simulink model "TV"  (R2025b)
settings: Solver=VariableStepAuto  StartTime=0.0  StopTime=10.0  RelTol=1e-3
undefined symbols (not defined in the file): tv
Description:
  | Adapted De Novellis et al. (IEEE TVT 2014) feedforward + PID TV controller.
settings Model: Creator=jaiden  LastModifiedBy=jaiden

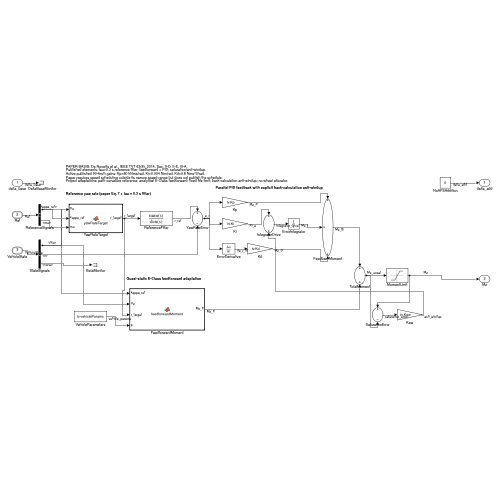
[thumbnail: Simulink's stored preview of the top-level diagram]
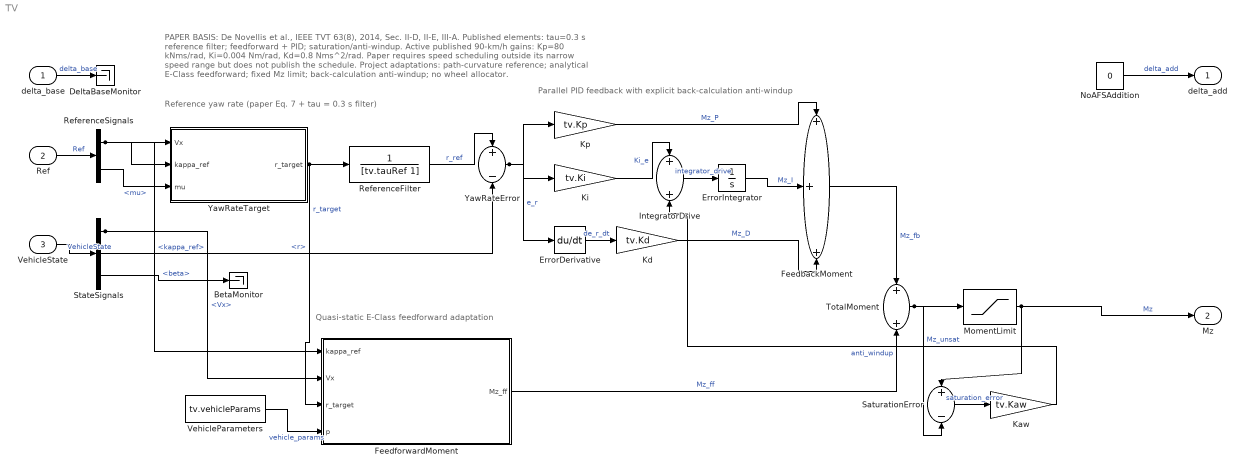
== system TV ==
  note: PAPER BASIS: De Novellis et al., IEEE TVT 63(8), 2014, Sec. II-D, II-E, III-A.
      | Published elements: tau=0.3 s reference filter; feedforward + PID; saturation/anti-windup.
      | Active published 90-km/h gains: Kp=80 kNms/rad, Ki=0.004 Nm/rad, Kd=0.8 Nms^2/rad.
      | Paper requires speed scheduling outside its narrow speed range but does not publish the schedule.
      | Project adaptations: path-curvature reference; analytical E-Class feedforward; fixed Mz limit; back-calculation anti-windup; no wheel allocator.
  note: Reference yaw rate (paper Eq. 7 + tau = 0.3 s filter)
  note: Parallel PID feedback with explicit back-calculation anti-windup
  note: Quasi-static E-Class feedforward adaptation
  delta_base : Inport
  Ref : Inport  Port=2  OutDataTypeStr=Bus: ReferenceBus
  VehicleState : Inport  Port=3  OutDataTypeStr=Bus: VehicleStateBus
  BetaMonitor : Terminator
  DeltaBaseMonitor : Terminator
  ErrorDerivative : Derivative
  ErrorIntegrator : Integrator
  FeedbackMoment : Sum  Inputs=+++
  FeedforwardMoment : MATLAB Function  TreatAsAtomicUnit=on
  IntegratorDrive : Sum  Description=Integral drive = Ki*e_r + Kaw*(Mz-Mz_unsat). The paper states
  Kaw : Gain  Description=Project-specific back-calculation gain. The paper confirms  Gain=tv.Kaw
  Kd : Gain  Gain=tv.Kd
  Ki : Gain  Gain=tv.Ki
  Kp : Gain  Gain=tv.Kp
  MomentLimit : Saturate  Description=Fixed bicycle-model yaw-moment authority; replace with plant-specific  UpperLimit=tv.MzMax  LowerLimit=-tv.MzMax  ZeroCross=off
  NoAFSAddition : Constant  Value=0
  ReferenceFilter : TransferFcn  Description=Paper Sec. II-D: first-order reference-yaw-rate factor, tau = 0.3 s.  Numerator=1  Denominator=[tv.tauRef 1]
  ReferenceSignals : BusSelector  OutputSignals=kappa_ref,mu
  SaturationError : Sum  Inputs=+-
  StateSignals : BusSelector  OutputSignals=Vx,r,beta
  TotalMoment : Sum
  VehicleParameters : Constant  Description=[m, a, b, Caf, Car] for analytical E-Class feedforward.  Value=tv.vehicleParams
  YawRateError : Sum  Description=e_r = r_ref - r matches negative feedback in paper Eq. (5) and  Inputs=+-
  YawRateTarget : MATLAB Function  TreatAsAtomicUnit=on
  delta_add : Outport
  Mz : Outport  Port=2
  wires:
  NoAFSAddition/1 -> delta_add/1  "delta_add"
  delta_base/1 -> DeltaBaseMonitor/1  "delta_base"
  Ref/1 -> ReferenceSignals/1  "Ref"
  VehicleState/1 -> StateSignals/1  "VehicleState"
  StateSignals/3 -> BetaMonitor/1  "<beta>"
  ReferenceSignals/1 -> YawRateTarget/2(kappa_ref), FeedforwardMoment/1(kappa_ref)  "<kappa_ref>"
  ReferenceSignals/2 -> YawRateTarget/3(mu)  "<mu>"
  StateSignals/1 -> YawRateTarget/1(Vx), FeedforwardMoment/2(Vx)  "<Vx>"
  YawRateTarget/1(r_target) -> ReferenceFilter/1, FeedforwardMoment/3(r_target)  "r_target"
  ReferenceFilter/1 -> YawRateError/1  "r_ref"
  StateSignals/2 -> YawRateError/2  "<r>"
  YawRateError/1 -> Kp/1, Ki/1, ErrorDerivative/1  "e_r"
  Ki/1 -> IntegratorDrive/1  "Ki_e"
  IntegratorDrive/1 -> ErrorIntegrator/1  "integrator_drive"
  ErrorDerivative/1 -> Kd/1  "de_r_dt"
  Kp/1 -> FeedbackMoment/1  "Mz_P"
  ErrorIntegrator/1 -> FeedbackMoment/2  "Mz_I"
  Kd/1 -> FeedbackMoment/3  "Mz_D"
  VehicleParameters/1 -> FeedforwardMoment/4(p)  "vehicle_params"
  FeedbackMoment/1 -> TotalMoment/1  "Mz_fb"
  FeedforwardMoment/1(Mz_ff) -> TotalMoment/2  "Mz_ff"
  TotalMoment/1 -> MomentLimit/1, SaturationError/2  "Mz_unsat"
  MomentLimit/1 -> Mz/1, SaturationError/1  "Mz"
  SaturationError/1 -> Kaw/1  "saturation_error"
  Kaw/1 -> IntegratorDrive/2  "anti_windup"

== matlab function TV/FeedforwardMoment ==
  data: kappa_ref input; Mz_ff output; Vx input; r_target input; p input
function Mz_ff = feedforwardMoment(kappa_ref, Vx, r_target, p)
%FEEDFORWARDMOMENT Analytical replacement for paper lookup tables.
% De Novellis Sec. III-A obtains Mz_ff from optimized quasi-static
% maps indexed by an exogenous driver steering demand. In this project
% the exogenous command is path curvature; delta_base also contains
% closed-loop path-error correction and is therefore not equivalent to
% the paper's driver input. Nominal kinematic steering is used instead.
%
% The unavailable maps are replaced by the same steady-equilibrium
% idea evaluated explicitly with the project linear bicycle model.
m = p(1); a = p(2); b = p(3); Caf = p(4); Car = p(5);
if abs(Vx) < 0.1
    Mz_ff = 0;
    return;
end
delta_nom = atan((a+b)*kappa_ref);
Vy_ss = (Caf*Vx*delta_nom + (b*Car-a*Caf)*r_target ...
         - m*Vx^2*r_target)/(Caf+Car);
alpha_f = delta_nom - (Vy_ss+a*r_target)/Vx;
alpha_r = -(Vy_ss-b*r_target)/Vx;
Fyf_ss = Caf*alpha_f;
Fyr_ss = Car*alpha_r;
% Enforce steady yaw equilibrium: 0 = a*Fyf-b*Fyr+Mz_ff.
Mz_ff = -(a*Fyf_ss-b*Fyr_ss);
end

== matlab function TV/YawRateTarget ==
  data: Vx input; r_target output; kappa_ref input; mu input
function r_target = yawRateTarget(Vx, kappa_ref, mu)
%YAWRATETARGET Path-based adaptation of De Novellis Sec. II-D.
% The paper uses r_ref,S = ay/V (Eq. 7). For a path with curvature
% kappa, ay = Vx^2*kappa, hence r_target = Vx*kappa.
%
% The paper's unavailable mu-dependent lookup table is represented
% here by the transparent physical bound |Vx*r| <= mu*g.
g = 9.81;
if abs(Vx) < 0.1
    % Numerical domain guard at standstill; inactive in test cases.
    r_target = 0;
    return;
end
r_path = Vx*kappa_ref;
r_limit = mu*g/abs(Vx);
r_target = min(max(r_path, -r_limit), r_limit);
end
